simulink model "LoFT_Example3"  (R2024b)
settings: Solver=ode4  StartTime=0.0  StopTime=300  FixedStep=simu.dt  RelTol=1e-3
undefined symbols (not defined in the file): body, circtime, Communication, D1, Delta, irkb, line, LoFT, p0, Pn, s, simu, trip_time, Turbwind, waves, wind
libraries: simulink x350, spsThreePhaseVIMeasurementLib x41, spsThreePhasePISectionLineLib x34, spsThreePhaseParallelRLCLoadLib x21, spsThreePhaseTransformerTwoWindingsLib x14, spsLoadFlowBusLib x10, spsThreePhaseDynamicLoadLib x9, spsSynchronousMachinepuStandardLib x7, spsExcitationSystemLib x7, spsSteamTurbineandGovernorLib x7, spsGenericPowerSystemStabilizerLib x7, spsMultiBandPowerSystemStabilizerLib x7
(part 38 of 49)

== system LoFT_Example3/FOWT System/Subsystem7/FOWT8/Hydrodynamics/excitation force ==
  position : Inport
  Wave : Inport  Port=2
  Clock : Clock  Commented=on
  Frequency Spacing Delta Omega : Constant  Commented=on  Value=waves.dOmega/10  VectorParams1D=off
  Imaginary Part of Wave Excitation : Constant  Commented=on  Value=body.hydroForce.fExt.im(:,:,[1,3,5])  VectorParams1D=off
  Random Phase : Constant  Commented=on  Value=waves.phase  VectorParams1D=off
  Real Part of Wave Excitation : Constant  Commented=on  Value=body.hydroForce.fExt.re(:,:,[1,3,5])  VectorParams1D=off
  Real Part of Wave Excitation1 : Constant  Commented=on  Value=body.hydroForce.fExt.md(:,:,[1,3,5])  VectorParams1D=off
  WECSim Linear wave excitiation : MATLAB Function  Commented=on  TreatAsAtomicUnit=on
  Wave Frequency : Constant  Commented=on  Value=waves.omega/10  VectorParams1D=off
  Wave Spectrum : Constant  Commented=on  Value=waves.amplitude  VectorParams1D=off
  Wave direction spread : Constant  Commented=on  Value=waves.spread  VectorParams1D=off
  Wave direction1 : Constant  Commented=on  Value=waves.direction  VectorParams1D=off
  Fext : Outport
  wires:
  Wave/1 -> Fext/1
  Wave direction1/1 -> WECSim Linear wave excitiation/8(WaveDir)
  Frequency Spacing Delta Omega/1 -> WECSim Linear wave excitiation/6(dw)
  Wave Spectrum/1 -> WECSim Linear wave excitiation/1(A)
  Imaginary Part of Wave Excitation/1 -> WECSim Linear wave excitiation/4(fExtIM)
  Random Phase/1 -> WECSim Linear wave excitiation/5(phaseRand)
  Wave Frequency/1 -> WECSim Linear wave excitiation/2(w)
  Real Part of Wave Excitation1/1 -> WECSim Linear wave excitiation/10(fExtMD)
  Wave direction spread/1 -> WECSim Linear wave excitiation/9(spread)
  Clock/1 -> WECSim Linear wave excitiation/7(time)
  Real Part of Wave Excitation/1 -> WECSim Linear wave excitiation/3(fExtRE)

== system LoFT_Example3/FOWT System/Subsystem7/FOWT8/Hydrodynamics/radiation force ==
  velocity : Inport
  In2 : Inport  Port=2
  Add : Sum
  Constant1 : Constant  Value=Hydro.radiationaddedmass
  Constant2 : Constant  Value=Hydro.radiationdamping
  Demux : Demux  Commented=on  Outputs=3
  Demux1 : Demux  Commented=on  Outputs=3
  Gain : Gain  Commented=on  Gain=-1
  IRBK : Constant  Commented=on  Value=irkb(:,[1,3,5],[[1,3,5]])
  MATLAB Function : MATLAB Function  Commented=on  TreatAsAtomicUnit=on
  Product : Product  Multiplication=Matrix(*)
  Product1 : Product  Multiplication=Matrix(*)
  Rate Transition : RateTransition  Commented=on
  Reshape : Reshape  Commented=on
  Scope1 : Scope  Commented=on  NumInputPorts=2
  Scope2 : Scope  Commented=on  NumInputPorts=2
  Scope3 : Scope  Commented=on  NumInputPorts=2
  cicTime : Constant  Commented=on  Value=circtime
  F_rad : Outport
  wires:
  Add/1 -> F_rad/1
  Product/1 -> Add/1
  Constant2/1 -> Product1/1
  Constant1/1 -> Product/1
  In2/1 -> MATLAB Function/1(velocity), Product1/2
  IRBK/1 -> MATLAB Function/2(irkb)
  Rate Transition/1 -> Reshape/1
  cicTime/1 -> MATLAB Function/3(circtime)
  MATLAB Function/1(radiationdamping) -> Rate Transition/1
  velocity/1 -> Product/2
  Reshape/1 -> Gain/1
  Demux1/1 -> Scope1/1
  Demux/1 -> Scope1/2
  Demux1/2 -> Scope2/1
  Demux/2 -> Scope2/2
  Demux1/3 -> Scope3/1
  Demux/3 -> Scope3/2
  Gain/1 -> Demux/1
  Product1/1 -> Demux1/1, Add/2

== system LoFT_Example3/FOWT System/Subsystem7/FOWT8/Hydrodynamics/viscous force  ==
  In1 : Inport
  Abs : Abs  SaturateOnIntegerOverflow=off
  Constant3 : Constant  Value=Hydro.viscious
  Product2 : Product  Multiplication=Matrix(*)
  Product3 : Product
  F_vis : Outport
  wires:
  Product2/1 -> F_vis/1
  Product3/1 -> Product2/2
  In1/1 -> Product3/2, Abs/1
  Constant3/1 -> Product2/1
  Abs/1 -> Product3/1

== system LoFT_Example3/FOWT System/Subsystem7/FOWT8/wind speed(m//s)/smooth1 ==
  In1 : Inport
  Gain : Gain
  Gain1 : Gain
  Integrator : Integrator
  Scope : Scope  NumInputPorts=2
  Sum : Sum  Inputs=|+-
  FB : Outport
  wires:
  Gain1/1 -> Scope/2, FB/1
  Integrator/1 -> Gain1/1, Gain/1
  Sum/1 -> Integrator/1
  Gain/1 -> Sum/2
  In1/1 -> Scope/1, Sum/1

== system LoFT_Example3/FOWT System/Subsystem7/FOWT9/Aerodynamics and Local Control Systems/Hull Aerodynamic ==
  In1 : Inport
  In2 : Inport  Port=2
  In4 : Inport  Port=3
  2-D Lookup Table1 : Lookup_n-D  BreakpointsForDimension1=Aero.TSR(1:1:24)  BreakpointsForDimension2=Aero.BlPitch(6:1:36)  Table=max(Aero.Ctmat(1:24,6:36),0)  InternalRulePriority=Speed  RndMeth=Simplest
      settings: InputPortMap=u0,u1
  Add1 : Sum
  Constant : Constant  Value=0
  Divide2 : Product  Inputs=*/
  Gain1 : Gain  Gain=0.5*1.225*pi*120^2*0.975*1.1
  Gain3 : Gain  Gain=120
  Gain5 : Gain  Gain=180/pi
  Product2 : Product
  Product3 : Product
  Saturation1 : Saturate  UpperLimit=2  LowerLimit=0
  Tower : Gain  Gain=0.613 * Aero.Cs * Aero.Ch * Aero.S
  Transfer Fcn2 : TransferFcn  Denominator=[0.2 1]
  Vector Concatenate1 : Concatenate  NumInputs=3
  mean force arm : Gain  Gain=92.8
  Out1 : Outport
  Rotor thrust : Outport  Port=2
  wires:
  Vector Concatenate1/1 -> Out1/1
  In4/1 -> Gain5/1
  In2/1 -> Gain3/1
  mean force arm/1 -> Vector Concatenate1/3
  Gain1/1 -> Product3/2
  Gain5/1 -> 2-D Lookup Table1/2
  Gain3/1 -> Divide2/1
  Divide2/1 -> 2-D Lookup Table1/1
  Product2/1 -> Product3/1, Tower/1
  Transfer Fcn2/1 -> Add1/2
  Constant/1 -> Vector Concatenate1/2
  Add1/1 -> mean force arm/1, Vector Concatenate1/1, Rotor thrust/1
  Saturation1/1 -> Gain1/1
  2-D Lookup Table1/1 -> Saturation1/1
  Product3/1 -> Transfer Fcn2/1
  In1/1 -> Divide2/2, Product2/1, Product2/2
  Tower/1 -> Add1/1

== system LoFT_Example3/FOWT System/Subsystem7/FOWT9/Aerodynamics and Local Control Systems/Local Control Systems ==
  WindSpeed : Inport
  RotSpeed : Inport  Port=2
  Nacelle Speed : Inport  Port=3
  " " : StateSpace  A=Controller.omegaFilter.A  B=Controller.omegaFilter.B  C=Controller.omegaFilter.C  D=Controller.omegaFilter.D  InitialCondition=[0,(7.55*pi/30)/Controller.omegaFilter.C(2)]
  Delay : Delay  DelayLength=1  InitialCondition=0
  Subsystem : Subsystem
  Subsystem1 : Subsystem
  Subsystem2 : Subsystem
  Transfer Fcn : TransferFcn  Denominator="[Controller.pitchFilter.A,   Controller.pitchFilter.B    1]"
  wind speed estimator : Subsystem
  GenTorq : Outport
  BldPitch : Outport  Port=2
  wires:
  wind speed estimator/1(Out1) -> Subsystem1/2(WindSpeed), Subsystem/1(WindSpeed)
  Delay/1 -> Subsystem1/3(3), Subsystem/2(2)
  [Delta_omega_g] -> Delay/1
  Subsystem/1(GenTorq) -> GenTorq/1, Subsystem2/1(GenTorq)
  Subsystem1/1(BldPitch) -> Subsystem2/2(BldPitch), BldPitch/1
  Subsystem2/1(Delta_omega_g) -> [Delta_omega_g]
  RotSpeed/1 -> " "/1
  Nacelle Speed/1 -> Transfer Fcn/1
  Transfer Fcn/1 -> Subsystem1/4(Nacelle Speed)
  " "/1 -> Subsystem1/1(RotSpeed), Subsystem/3(RotSpeed)
  WindSpeed/1 -> wind speed estimator/1(In1)

== system LoFT_Example3/FOWT System/Subsystem7/FOWT9/Aerodynamics and Local Control Systems/Rotor//drivetrain dynamics ==
  In1 : Inport
  In2 : Inport  Port=2
  In3 : Inport  Port=3
  In4 : Inport  Port=4
  In5 : Inport  Port=5
  1/J_rot : Gain  Gain=1/(LoFT.Property.rotorinertia)
  2-D Lookup Table : Lookup_n-D  BreakpointsForDimension1=Aero.TSR(1:1:24)  BreakpointsForDimension2=Aero.BlPitch(6:1:36)  Table=max(Aero.Cpmat(1:24,6:36),0)  InternalRulePriority=Speed  RndMeth=Simplest
      settings: InputPortMap=u0,u1
  Divide : Product  Inputs=**/
  Divide1 : Product  Inputs=*/
  Gain : Gain  Gain=0.5 * 1.225 * pi * 120^2 * 0.965 * 0.975
  Gain2 : Gain  Gain=120
  Gain4 : Gain  Gain=180/pi
  Integrator : Integrator  InitialCondition=Initstate(1)
  Product1 : Product  Inputs=3
  Saturation : Saturate  UpperLimit=1  LowerLimit=0
  Saturation3 : Saturate  UpperLimit=1.5  LowerLimit=0.3
  Sum : Sum  Inputs=|+-
  Transfer Fcn1 : TransferFcn  Denominator=[0.2 1]
  Out1 : Outport
  Out2 : Outport  Port=2
  wires:
  In1/1 -> Gain2/1
  In2/1 -> Divide1/2
  Sum/1 -> Transfer Fcn1/1
  In5/1 -> Sum/2
  Product1/1 -> Divide/2
  Gain2/1 -> Divide1/1
  Gain/1 -> Divide/1
  1/J_rot/1 -> Integrator/1
  Integrator/1 -> Saturation3/1
  In3/1 -> Gain4/1
  Transfer Fcn1/1 -> 1/J_rot/1
  2-D Lookup Table/1 -> Saturation/1
  Gain4/1 -> 2-D Lookup Table/2
  In4/1 -> Product1/1, Product1/2, Product1/3
  Saturation/1 -> Gain/1
  Divide1/1 -> 2-D Lookup Table/1
  Divide/1 -> Sum/1, Out2/1
  Saturation3/1 -> Divide/3, Out1/1

== system LoFT_Example3/FOWT System/Subsystem7/FOWT9/Aerodynamics and Local Control Systems/smooth1 ==
  In1 : Inport
  Gain : Gain  Gain=10
  Gain1 : Gain  Gain=10
  Integrator : Integrator  InitialCondition=0.1*8e6
  Scope : Scope  NumInputPorts=2
  Sum : Sum  Inputs=|+-
  Out1 : Outport
  wires:
  In1/1 -> Sum/1, Scope/1
  Gain/1 -> Sum/2
  Sum/1 -> Integrator/1
  Integrator/1 -> Gain/1, Gain1/1
  Gain1/1 -> Out1/1, Scope/2

== system LoFT_Example3/FOWT System/Subsystem7/FOWT9/Aerodynamics and Local Control Systems/wind speed estimator ==
  In1 : Inport
  Discrete Filter : DiscreteFilter  Numerator=Controller.F.Wind.b  Denominator=Controller.F.Wind.a  InitialStates=2000
  Out1 : Outport
  wires:
  Discrete Filter/1 -> Out1/1
  In1/1 -> Discrete Filter/1

== system LoFT_Example3/FOWT System/Subsystem7/FOWT9/Hydrodynamics/excitation force ==
  position : Inport
  Wave : Inport  Port=2
  Clock : Clock  Commented=on
  Frequency Spacing Delta Omega : Constant  Commented=on  Value=waves.dOmega/10  VectorParams1D=off
  Imaginary Part of Wave Excitation : Constant  Commented=on  Value=body.hydroForce.fExt.im(:,:,[1,3,5])  VectorParams1D=off
  Random Phase : Constant  Commented=on  Value=waves.phase  VectorParams1D=off
  Real Part of Wave Excitation : Constant  Commented=on  Value=body.hydroForce.fExt.re(:,:,[1,3,5])  VectorParams1D=off
  Real Part of Wave Excitation1 : Constant  Commented=on  Value=body.hydroForce.fExt.md(:,:,[1,3,5])  VectorParams1D=off
  WECSim Linear wave excitiation : MATLAB Function  Commented=on  TreatAsAtomicUnit=on
  Wave Frequency : Constant  Commented=on  Value=waves.omega/10  VectorParams1D=off
  Wave Spectrum : Constant  Commented=on  Value=waves.amplitude  VectorParams1D=off
  Wave direction spread : Constant  Commented=on  Value=waves.spread  VectorParams1D=off
  Wave direction1 : Constant  Commented=on  Value=waves.direction  VectorParams1D=off
  Fext : Outport
  wires:
  Real Part of Wave Excitation/1 -> WECSim Linear wave excitiation/3(fExtRE)
  Clock/1 -> WECSim Linear wave excitiation/7(time)
  Wave direction spread/1 -> WECSim Linear wave excitiation/9(spread)
  Real Part of Wave Excitation1/1 -> WECSim Linear wave excitiation/10(fExtMD)
  Wave Frequency/1 -> WECSim Linear wave excitiation/2(w)
  Random Phase/1 -> WECSim Linear wave excitiation/5(phaseRand)
  Imaginary Part of Wave Excitation/1 -> WECSim Linear wave excitiation/4(fExtIM)
  Wave Spectrum/1 -> WECSim Linear wave excitiation/1(A)
  Frequency Spacing Delta Omega/1 -> WECSim Linear wave excitiation/6(dw)
  Wave direction1/1 -> WECSim Linear wave excitiation/8(WaveDir)
  Wave/1 -> Fext/1

== system LoFT_Example3/FOWT System/Subsystem7/FOWT9/Hydrodynamics/radiation force ==
  velocity : Inport
  In2 : Inport  Port=2
  Add : Sum
  Constant1 : Constant  Value=Hydro.radiationaddedmass
  Constant2 : Constant  Value=Hydro.radiationdamping
  Demux : Demux  Commented=on  Outputs=3
  Demux1 : Demux  Commented=on  Outputs=3
  Gain : Gain  Commented=on  Gain=-1
  IRBK : Constant  Commented=on  Value=irkb(:,[1,3,5],[[1,3,5]])
  MATLAB Function : MATLAB Function  Commented=on  TreatAsAtomicUnit=on
  Product : Product  Multiplication=Matrix(*)
  Product1 : Product  Multiplication=Matrix(*)
  Rate Transition : RateTransition  Commented=on
  Reshape : Reshape  Commented=on
  Scope1 : Scope  Commented=on  NumInputPorts=2
  Scope2 : Scope  Commented=on  NumInputPorts=2
  Scope3 : Scope  Commented=on  NumInputPorts=2
  cicTime : Constant  Commented=on  Value=circtime
  F_rad : Outport
  wires:
  Product1/1 -> Add/2, Demux1/1
  Gain/1 -> Demux/1
  Demux/3 -> Scope3/2
  Demux1/3 -> Scope3/1
  Demux/2 -> Scope2/2
  Demux1/2 -> Scope2/1
  Demux/1 -> Scope1/2
  Demux1/1 -> Scope1/1
  Reshape/1 -> Gain/1
  velocity/1 -> Product/2
  MATLAB Function/1(radiationdamping) -> Rate Transition/1
  cicTime/1 -> MATLAB Function/3(circtime)
  Rate Transition/1 -> Reshape/1
  IRBK/1 -> MATLAB Function/2(irkb)
  In2/1 -> Product1/2, MATLAB Function/1(velocity)
  Constant1/1 -> Product/1
  Constant2/1 -> Product1/1
  Product/1 -> Add/1
  Add/1 -> F_rad/1

== system LoFT_Example3/FOWT System/Subsystem7/FOWT9/Hydrodynamics/viscous force  ==
  In1 : Inport
  Abs : Abs  SaturateOnIntegerOverflow=off
  Constant3 : Constant  Value=Hydro.viscious
  Product2 : Product  Multiplication=Matrix(*)
  Product3 : Product
  F_vis : Outport
  wires:
  Abs/1 -> Product3/1
  Constant3/1 -> Product2/1
  In1/1 -> Abs/1, Product3/2
  Product3/1 -> Product2/2
  Product2/1 -> F_vis/1

== system LoFT_Example3/FOWT System/Subsystem7/FOWT9/wind speed(m//s)/smooth1 ==
  In1 : Inport
  Gain : Gain
  Gain1 : Gain
  Integrator : Integrator
  Scope : Scope  NumInputPorts=2
  Sum : Sum  Inputs=|+-
  FB : Outport
  wires:
  In1/1 -> Sum/1, Scope/1
  Gain/1 -> Sum/2
  Sum/1 -> Integrator/1
  Integrator/1 -> Gain/1, Gain1/1
  Gain1/1 -> FB/1, Scope/2

== system LoFT_Example3/Onshore grid/Onshore Grid/Subsystem/SG1/Regulators1 ==
  m : Inport
  Bus Selector1 : BusSelector  OutputSignals="dq0 components.Stator voltage  vq (pu),dq0 components.Stator voltage  vd (pu),Mechanical.Rotor speed  wm  (pu),Output active power   Peo (pu)"
  Math Function1 : Math  Operator=hypot  SignedPower=on
  Pref1 : Constant
  Scope : Scope
  Turbine  & Excitation Regulators Mac2 : Subsystem
  Vref : Constant
  Pm : Outport  VectorParamsAs1DForOutWhenUnconnected=off
  Vf : Outport  Port=2  VectorParamsAs1DForOutWhenUnconnected=off
  wires:
  m/1 -> Bus Selector1/1
  Bus Selector1/4 -> Turbine  & Excitation Regulators Mac2/6(Pe)  "<Output active power   Peo (pu)>"
  Bus Selector1/3 -> Turbine  & Excitation Regulators Mac2/5(w)  "<Rotor speed  wm  (pu)>"
  Bus Selector1/2 -> Turbine  & Excitation Regulators Mac2/3(Vd), Math Function1/2  "<Stator voltage  vd (pu)>"
  Bus Selector1/1 -> Turbine  & Excitation Regulators Mac2/4(Vq), Math Function1/1  "<Stator voltage  vq (pu)>"
  Turbine  & Excitation Regulators Mac2/2(Vf) -> Vf/1
  Vref/1 -> Turbine  & Excitation Regulators Mac2/1(Pref)
  Turbine  & Excitation Regulators Mac2/1(Pm) -> Pm/1
  Pref1/1 -> Turbine  & Excitation Regulators Mac2/2(Vref)
  Math Function1/1 -> Scope/1

== system LoFT_Example3/Onshore grid/Onshore Grid/Subsystem/SG2/Regulators2 ==
  m : Inport
  Bus Selector1 : BusSelector  OutputSignals="dq0 components.Stator voltage  vq (pu),dq0 components.Stator voltage  vd (pu),Mechanical.Rotor speed  wm  (pu),Output active power   Peo (pu)"
  Math Function1 : Math  Operator=hypot  SignedPower=on
  Pref1 : Constant
  Scope : Scope
  Turbine  & Excitation Regulators Mac2 : Subsystem
  Vref : Constant  Value=0.52081
  Pm : Outport  VectorParamsAs1DForOutWhenUnconnected=off
  Vf : Outport  Port=2  VectorParamsAs1DForOutWhenUnconnected=off
  wires:
  m/1 -> Bus Selector1/1
  Bus Selector1/4 -> Turbine  & Excitation Regulators Mac2/6(Pe)  "<Output active power   Peo (pu)>"
  Bus Selector1/3 -> Turbine  & Excitation Regulators Mac2/5(w)  "<Rotor speed  wm  (pu)>"
  Bus Selector1/2 -> Turbine  & Excitation Regulators Mac2/3(Vd), Math Function1/2  "<Stator voltage  vd (pu)>"
  Bus Selector1/1 -> Turbine  & Excitation Regulators Mac2/4(Vq), Math Function1/1  "<Stator voltage  vq (pu)>"
  Turbine  & Excitation Regulators Mac2/2(Vf) -> Vf/1
  Vref/1 -> Turbine  & Excitation Regulators Mac2/1(Pref)
  Turbine  & Excitation Regulators Mac2/1(Pm) -> Pm/1
  Pref1/1 -> Turbine  & Excitation Regulators Mac2/2(Vref)
  Math Function1/1 -> Scope/1

== system LoFT_Example3/Onshore grid/Onshore Grid/Subsystem/SG4/Regulators4 ==
  m : Inport
  Bus Selector1 : BusSelector  OutputSignals="dq0 components.Stator voltage  vq (pu),dq0 components.Stator voltage  vd (pu),Mechanical.Rotor speed  wm  (pu),Output active power   Peo (pu)"
  Math Function1 : Math  Operator=hypot  SignedPower=on
  Pref1 : Constant
  Scope : Scope
  Turbine  & Excitation Regulators Mac2 : Subsystem
  Vref : Constant  Value=0.632
  Pm : Outport  VectorParamsAs1DForOutWhenUnconnected=off
  Vf : Outport  Port=2  VectorParamsAs1DForOutWhenUnconnected=off
  wires:
  m/1 -> Bus Selector1/1
  Bus Selector1/4 -> Turbine  & Excitation Regulators Mac2/6(Pe)  "<Output active power   Peo (pu)>"
  Bus Selector1/3 -> Turbine  & Excitation Regulators Mac2/5(w)  "<Rotor speed  wm  (pu)>"
  Bus Selector1/2 -> Turbine  & Excitation Regulators Mac2/3(Vd), Math Function1/2  "<Stator voltage  vd (pu)>"
  Bus Selector1/1 -> Turbine  & Excitation Regulators Mac2/4(Vq), Math Function1/1  "<Stator voltage  vq (pu)>"
  Turbine  & Excitation Regulators Mac2/2(Vf) -> Vf/1
  Vref/1 -> Turbine  & Excitation Regulators Mac2/1(Pref)
  Turbine  & Excitation Regulators Mac2/1(Pm) -> Pm/1
  Pref1/1 -> Turbine  & Excitation Regulators Mac2/2(Vref)
  Math Function1/1 -> Scope/1

== system LoFT_Example3/Onshore grid/Onshore Grid/Subsystem/SG5/Regulators5 ==
  m : Inport
  Bus Selector1 : BusSelector  OutputSignals="dq0 components.Stator voltage  vq (pu),dq0 components.Stator voltage  vd (pu),Mechanical.Rotor speed  wm  (pu),Output active power   Peo (pu)"
  Math Function1 : Math  Operator=hypot  SignedPower=on
  Pref1 : Constant
  Scope : Scope
  Turbine  & Excitation Regulators Mac2 : Subsystem
  Vref : Constant  Value=0.508
  Pm : Outport  VectorParamsAs1DForOutWhenUnconnected=off
  Vf : Outport  Port=2  VectorParamsAs1DForOutWhenUnconnected=off
  wires:
  m/1 -> Bus Selector1/1
  Bus Selector1/4 -> Turbine  & Excitation Regulators Mac2/6(Pe)  "<Output active power   Peo (pu)>"
  Bus Selector1/3 -> Turbine  & Excitation Regulators Mac2/5(w)  "<Rotor speed  wm  (pu)>"
  Math Function1/1 -> Scope/1
  Bus Selector1/2 -> Turbine  & Excitation Regulators Mac2/3(Vd), Math Function1/2  "<Stator voltage  vd (pu)>"
  Bus Selector1/1 -> Turbine  & Excitation Regulators Mac2/4(Vq), Math Function1/1  "<Stator voltage  vq (pu)>"
  Turbine  & Excitation Regulators Mac2/2(Vf) -> Vf/1
  Vref/1 -> Turbine  & Excitation Regulators Mac2/1(Pref)
  Turbine  & Excitation Regulators Mac2/1(Pm) -> Pm/1
  Pref1/1 -> Turbine  & Excitation Regulators Mac2/2(Vref)

== system LoFT_Example3/Onshore grid/Onshore Grid/Subsystem/SG6/Regulators6 ==
  m : Inport
  Bus Selector1 : BusSelector  OutputSignals="dq0 components.Stator voltage  vq (pu),dq0 components.Stator voltage  vd (pu),Mechanical.Rotor speed  wm  (pu),Output active power   Peo (pu)"
  Math Function1 : Math  Operator=hypot  SignedPower=on
  Pref1 : Constant
  Scope : Scope
  Turbine  & Excitation Regulators Mac2 : Subsystem
  Vref : Constant  Value=0.65
  Pm : Outport  VectorParamsAs1DForOutWhenUnconnected=off
  Vf : Outport  Port=2  VectorParamsAs1DForOutWhenUnconnected=off
  wires:
  m/1 -> Bus Selector1/1
  Bus Selector1/4 -> Turbine  & Excitation Regulators Mac2/6(Pe)  "<Output active power   Peo (pu)>"
  Bus Selector1/3 -> Turbine  & Excitation Regulators Mac2/5(w)  "<Rotor speed  wm  (pu)>"
  Bus Selector1/2 -> Turbine  & Excitation Regulators Mac2/3(Vd), Math Function1/2  "<Stator voltage  vd (pu)>"
  Bus Selector1/1 -> Turbine  & Excitation Regulators Mac2/4(Vq), Math Function1/1  "<Stator voltage  vq (pu)>"
  Turbine  & Excitation Regulators Mac2/2(Vf) -> Vf/1
  Vref/1 -> Turbine  & Excitation Regulators Mac2/1(Pref)
  Turbine  & Excitation Regulators Mac2/1(Pm) -> Pm/1
  Pref1/1 -> Turbine  & Excitation Regulators Mac2/2(Vref)
  Math Function1/1 -> Scope/1

== system LoFT_Example3/Onshore grid/Onshore Grid/Subsystem/SG8/Regulators8 ==
  m : Inport
  Bus Selector1 : BusSelector  OutputSignals="dq0 components.Stator voltage  vq (pu),dq0 components.Stator voltage  vd (pu),Mechanical.Rotor speed  wm  (pu),Output active power   Peo (pu)"
  Math Function1 : Math  Operator=hypot  SignedPower=on
  Pref1 : Constant
  Scope : Scope
  Turbine  & Excitation Regulators Mac2 : Subsystem
  Vref : Constant  Value=0.54
  Pm : Outport  VectorParamsAs1DForOutWhenUnconnected=off
  Vf : Outport  Port=2  VectorParamsAs1DForOutWhenUnconnected=off
  wires:
  m/1 -> Bus Selector1/1
  Bus Selector1/4 -> Turbine  & Excitation Regulators Mac2/6(Pe)  "<Output active power   Peo (pu)>"
  Bus Selector1/3 -> Turbine  & Excitation Regulators Mac2/5(w)  "<Rotor speed  wm  (pu)>"
  Bus Selector1/2 -> Turbine  & Excitation Regulators Mac2/3(Vd), Math Function1/2  "<Stator voltage  vd (pu)>"
  Bus Selector1/1 -> Turbine  & Excitation Regulators Mac2/4(Vq), Math Function1/1  "<Stator voltage  vq (pu)>"
  Turbine  & Excitation Regulators Mac2/2(Vf) -> Vf/1
  Vref/1 -> Turbine  & Excitation Regulators Mac2/1(Pref)
  Turbine  & Excitation Regulators Mac2/1(Pm) -> Pm/1
  Pref1/1 -> Turbine  & Excitation Regulators Mac2/2(Vref)
  Math Function1/1 -> Scope/1

== system LoFT_Example3/Onshore grid/Onshore Grid/Subsystem/SG9/Regulators9 ==
  m : Inport
  Bus Selector1 : BusSelector  OutputSignals="dq0 components.Stator voltage  vq (pu),dq0 components.Stator voltage  vd (pu),Mechanical.Rotor speed  wm  (pu),Output active power   Peo (pu)"
  Math Function1 : Math  Operator=hypot  SignedPower=on
  Pref1 : Constant
  Scope : Scope
  Turbine  & Excitation Regulators Mac2 : Subsystem
  Vref : Constant  Value=0.83
  Pm : Outport  VectorParamsAs1DForOutWhenUnconnected=off
  Vf : Outport  Port=2  VectorParamsAs1DForOutWhenUnconnected=off
  wires:
  m/1 -> Bus Selector1/1
  Bus Selector1/4 -> Turbine  & Excitation Regulators Mac2/6(Pe)  "<Output active power   Peo (pu)>"
  Bus Selector1/3 -> Turbine  & Excitation Regulators Mac2/5(w)  "<Rotor speed  wm  (pu)>"
  Bus Selector1/2 -> Turbine  & Excitation Regulators Mac2/3(Vd), Math Function1/2  "<Stator voltage  vd (pu)>"
  Bus Selector1/1 -> Turbine  & Excitation Regulators Mac2/4(Vq), Math Function1/1  "<Stator voltage  vq (pu)>"
  Turbine  & Excitation Regulators Mac2/2(Vf) -> Vf/1
  Vref/1 -> Turbine  & Excitation Regulators Mac2/1(Pref)
  Turbine  & Excitation Regulators Mac2/1(Pm) -> Pm/1
  Pref1/1 -> Turbine  & Excitation Regulators Mac2/2(Vref)
  Math Function1/1 -> Scope/1

== system LoFT_Example3/FOWT System/Subsystem1/FOWT1/Aerodynamics and Local Control Systems/Local Control Systems/Subsystem ==
  WindSpeed : Inport
  2 : Inport  Port=2
  RotSpeed : Inport  Port=3
  Compare To Constant1 : simulink/Logic and Bit Operations/Compare To Constant  relop=>=  const=0  OutDataTypeStr=boolean
  Divide4 : Product  Inputs=**
  Gain5 : Gain  Gain=Controller.R.VS_KI
  Gain6 : Gain  Gain=Controller.R.VS_KP
  Integrator1 : Integrator  InitialCondition=Controller.torqueMax * 0.7  LimitOutput=on  UpperSaturationLimit=Controller.torqueMax
  Optimall TSR / Radius : Gain  Gain=Controller.R.VS_TSRopt/Controller.R.RotorRad
  Rate Limiter : RateLimiter  RisingSlewLimit=Controller.torqueMaxRate  FallingSlewLimit=-Controller.torqueMaxRate  SampleTimeMode=inherited
  Saturation : Saturate  UpperLimit=7.55*pi/30  LowerLimit=5*pi/30
  Saturation1 : Saturate  UpperLimit=Controller.torqueMax  LowerLimit=0
  Saturation2 : Saturate  UpperLimit=7.55*pi/30  LowerLimit=5*pi/30
  Scope2 : Scope
  Sum2 : Sum  Inputs=|+-
  Sum7 : Sum  Inputs=|+-
  Sum8 : Sum  Inputs=|++
  GenTorq : Outport
  wires:
  Gain6/1 -> Sum8/1
  WindSpeed/1 -> Optimall TSR / Radius/1
  Sum7/1 -> Saturation/1
  Divide4/1 -> Scope2/1, Sum7/2
  2/1 -> Compare To Constant1/1, Divide4/2
  Rate Limiter/1 -> GenTorq/1
  Saturation/1 -> Sum2/1
  Compare To Constant1/1 -> Divide4/1
  Sum2/1 -> Gain6/1, Gain5/1
  Integrator1/1 -> Sum8/2
  Gain5/1 -> Integrator1/1
  Sum8/1 -> Saturation1/1
  RotSpeed/1 -> Sum2/2
  Saturation1/1 -> Rate Limiter/1
  Saturation2/1 -> Sum7/1
  Optimall TSR / Radius/1 -> Saturation2/1

== system LoFT_Example3/FOWT System/Subsystem1/FOWT1/Aerodynamics and Local Control Systems/Local Control Systems/Subsystem1 ==
  RotSpeed : Inport
  WindSpeed : Inport  Port=2
  3 : Inport  Port=3
  Nacelle Speed : Inport  Port=4
  1-D Lookup Table : Lookup_n-D  NumberOfTableDimensions=1  BreakpointsForDimension1=Controller.R.PS_WindSpeeds  Table=Controller.R.PS_BldPitchMin  InternalRulePriority=Speed  RndMeth=Simplest
  Compare To Constant : simulink/Logic and Bit Operations/Compare To Constant  relop=<=  const=0  OutDataTypeStr=boolean
  Constant : Constant  Value=7.55*pi/30
  Constant1 : Constant  Value=90*pi/180
  Delay : Delay  DelayLength=1  InitialCondition=0
  Divide3 : Product  Inputs=**
  Gain : Gain  Gain=Controller.KV *0.5
  Gain Scheduling : Subsystem
  Gain1 : Gain
  Rate Limiter : RateLimiter  RisingSlewLimit=2*pi/180  FallingSlewLimit=-2 * pi/180  SampleTimeMode=inherited
  Saturation : Saturate  UpperLimit=7.55*pi/30  LowerLimit=5*pi/30
  Saturation Dynamic : simulink/Discontinuities/Saturation Dynamic  OutMin=[]  OutMax=[]  OutDataTypeStr=Inherit: Same as second input  OutDataType=fixdt(1, 16)  OutScaling=2^-10  DoSatur=off
  Scope2 : Scope
  Sum1 : Sum  Inputs=|++
  Sum3 : Sum  Inputs=|+-
  Sum4 : Sum  Inputs=|+-
  BldPitch : Outport
  wires:
  Saturation/1 -> Sum3/1
  Sum4/1 -> Saturation/1
  Rate Limiter/1 -> BldPitch/1
  Gain1/1 -> Scope2/1, Gain Scheduling/2(In3), Saturation Dynamic/3
  1-D Lookup Table/1 -> Gain1/1
  WindSpeed/1 -> 1-D Lookup Table/1  "Vhat"
  Nacelle Speed/1 -> Gain/1
  Gain/1 -> Sum1/2
  Sum1/1 -> Saturation Dynamic/2
  Gain Scheduling/1(Out1) -> Sum1/1
  RotSpeed/1 -> Sum3/2
  Delay/1 -> Gain Scheduling/3(In2)
  3/1 -> Divide3/2, Compare To Constant/1
  Constant1/1 -> Saturation Dynamic/1
  Constant/1 -> Sum4/1
  Compare To Constant/1 -> Divide3/1
  Saturation Dynamic/1 -> Delay/1, Rate Limiter/1
  Sum3/1 -> Gain Scheduling/1(In1)
  Divide3/1 -> Sum4/2

== system LoFT_Example3/FOWT System/Subsystem1/FOWT1/Aerodynamics and Local Control Systems/Local Control Systems/Subsystem2 ==
  GenTorq : Inport
  BldPitch : Inport  Port=2
  Constant3 : Constant  Value=-Controller.torqueMax
  Gain 1 : Gain  Gain=Controller.SPS_kb/deg2rad(30)
  Gain 2 : Gain  Gain=Controller.omegaMax
  Gain 3 : Gain  Gain=-Controller.SPS_kt/Controller.torqueMax
  Sum5 : Sum  Inputs=|+-
  Sum6 : Sum  Inputs=|+-
  Delta_omega_g : Outport
  wires:
  GenTorq/1 -> Sum5/1
  BldPitch/1 -> Gain 1/1
  Gain 2/1 -> Delta_omega_g/1
  Sum5/1 -> Gain 3/1
  Gain 3/1 -> Sum6/2
  Constant3/1 -> Sum5/2
  Gain 1/1 -> Sum6/1
  Sum6/1 -> Gain 2/1

== system LoFT_Example3/FOWT System/Subsystem1/FOWT1/Aerodynamics and Local Control Systems/Local Control Systems/wind speed estimator ==
  In1 : Inport
  Discrete Filter : DiscreteFilter  Numerator=Controller.F.Wind.b  Denominator=Controller.F.Wind.a  InitialStates=2000
  Out1 : Outport
  wires:
  In1/1 -> Discrete Filter/1
  Discrete Filter/1 -> Out1/1

== system LoFT_Example3/FOWT System/Subsystem1/FOWT10/Aerodynamics and Local Control Systems/Local Control Systems/Subsystem ==
  WindSpeed : Inport
  2 : Inport  Port=2
  RotSpeed : Inport  Port=3
  Compare To Constant1 : simulink/Logic and Bit Operations/Compare To Constant  relop=>=  const=0  OutDataTypeStr=boolean
  Divide4 : Product  Inputs=**
  Gain5 : Gain  Gain=Controller.R.VS_KI
  Gain6 : Gain  Gain=Controller.R.VS_KP
  Integrator1 : Integrator  InitialCondition=Controller.torqueMax * 0.7  LimitOutput=on  UpperSaturationLimit=Controller.torqueMax
  Optimall TSR / Radius : Gain  Gain=Controller.R.VS_TSRopt/Controller.R.RotorRad
  Rate Limiter : RateLimiter  RisingSlewLimit=Controller.torqueMaxRate  FallingSlewLimit=-Controller.torqueMaxRate  SampleTimeMode=inherited
  Saturation : Saturate  UpperLimit=7.55*pi/30  LowerLimit=5*pi/30
  Saturation1 : Saturate  UpperLimit=Controller.torqueMax  LowerLimit=0
  Saturation2 : Saturate  UpperLimit=7.55*pi/30  LowerLimit=5*pi/30
  Scope2 : Scope
  Sum2 : Sum  Inputs=|+-
  Sum7 : Sum  Inputs=|+-
  Sum8 : Sum  Inputs=|++
  GenTorq : Outport
  wires:
  Optimall TSR / Radius/1 -> Saturation2/1
  Saturation2/1 -> Sum7/1
  Saturation1/1 -> Rate Limiter/1
  RotSpeed/1 -> Sum2/2
  Sum8/1 -> Saturation1/1
  Gain5/1 -> Integrator1/1
  Integrator1/1 -> Sum8/2
  Sum2/1 -> Gain5/1, Gain6/1
  Compare To Constant1/1 -> Divide4/1
  Saturation/1 -> Sum2/1
  Rate Limiter/1 -> GenTorq/1
  2/1 -> Divide4/2, Compare To Constant1/1
  Divide4/1 -> Sum7/2, Scope2/1
  Sum7/1 -> Saturation/1
  WindSpeed/1 -> Optimall TSR / Radius/1
  Gain6/1 -> Sum8/1

== system LoFT_Example3/FOWT System/Subsystem1/FOWT10/Aerodynamics and Local Control Systems/Local Control Systems/Subsystem1 ==
  RotSpeed : Inport
  WindSpeed : Inport  Port=2
  3 : Inport  Port=3
  Nacelle Speed : Inport  Port=4
  1-D Lookup Table : Lookup_n-D  NumberOfTableDimensions=1  BreakpointsForDimension1=Controller.R.PS_WindSpeeds  Table=Controller.R.PS_BldPitchMin  InternalRulePriority=Speed  RndMeth=Simplest
  Compare To Constant : simulink/Logic and Bit Operations/Compare To Constant  relop=<=  const=0  OutDataTypeStr=boolean
  Constant : Constant  Value=7.55*pi/30
  Constant1 : Constant  Value=90*pi/180
  Delay : Delay  DelayLength=1  InitialCondition=0
  Divide3 : Product  Inputs=**
  Gain : Gain  Gain=Controller.KV *0.5
  Gain Scheduling : Subsystem
  Gain1 : Gain
  Rate Limiter : RateLimiter  RisingSlewLimit=2*pi/180  FallingSlewLimit=-2 * pi/180  SampleTimeMode=inherited
  Saturation : Saturate  UpperLimit=7.55*pi/30  LowerLimit=5*pi/30
  Saturation Dynamic : simulink/Discontinuities/Saturation Dynamic  OutMin=[]  OutMax=[]  OutDataTypeStr=Inherit: Same as second input  OutDataType=fixdt(1, 16)  OutScaling=2^-10  DoSatur=off
  Scope2 : Scope
  Sum1 : Sum  Inputs=|++
  Sum3 : Sum  Inputs=|+-
  Sum4 : Sum  Inputs=|+-
  BldPitch : Outport
  wires:
  Divide3/1 -> Sum4/2
  Sum3/1 -> Gain Scheduling/1(In1)
  Saturation Dynamic/1 -> Rate Limiter/1, Delay/1
  Compare To Constant/1 -> Divide3/1
  Constant/1 -> Sum4/1
  Constant1/1 -> Saturation Dynamic/1
  3/1 -> Compare To Constant/1, Divide3/2
  Delay/1 -> Gain Scheduling/3(In2)
  RotSpeed/1 -> Sum3/2
  Gain Scheduling/1(Out1) -> Sum1/1
  Sum1/1 -> Saturation Dynamic/2
  Gain/1 -> Sum1/2
  Nacelle Speed/1 -> Gain/1
  WindSpeed/1 -> 1-D Lookup Table/1  "Vhat"
  1-D Lookup Table/1 -> Gain1/1
  Gain1/1 -> Saturation Dynamic/3, Gain Scheduling/2(In3), Scope2/1
  Rate Limiter/1 -> BldPitch/1
  Sum4/1 -> Saturation/1
  Saturation/1 -> Sum3/1

== system LoFT_Example3/FOWT System/Subsystem1/FOWT10/Aerodynamics and Local Control Systems/Local Control Systems/Subsystem2 ==
  GenTorq : Inport
  BldPitch : Inport  Port=2
  Constant3 : Constant  Value=-Controller.torqueMax
  Gain 1 : Gain  Gain=Controller.SPS_kb/deg2rad(30)
  Gain 2 : Gain  Gain=Controller.omegaMax
  Gain 3 : Gain  Gain=-Controller.SPS_kt/Controller.torqueMax
  Sum5 : Sum  Inputs=|+-
  Sum6 : Sum  Inputs=|+-
  Delta_omega_g : Outport
  wires:
  Sum6/1 -> Gain 2/1
  Gain 1/1 -> Sum6/1
  Constant3/1 -> Sum5/2
  Gain 3/1 -> Sum6/2
  Sum5/1 -> Gain 3/1
  Gain 2/1 -> Delta_omega_g/1
  BldPitch/1 -> Gain 1/1
  GenTorq/1 -> Sum5/1

== system LoFT_Example3/FOWT System/Subsystem1/FOWT10/Aerodynamics and Local Control Systems/Local Control Systems/wind speed estimator ==
  In1 : Inport
  Discrete Filter : DiscreteFilter  Numerator=Controller.F.Wind.b  Denominator=Controller.F.Wind.a  InitialStates=2000
  Out1 : Outport
  wires:
  Discrete Filter/1 -> Out1/1
  In1/1 -> Discrete Filter/1

== system LoFT_Example3/FOWT System/Subsystem1/FOWT2/Aerodynamics and Local Control Systems/Local Control Systems/Subsystem ==
  WindSpeed : Inport
  2 : Inport  Port=2
  RotSpeed : Inport  Port=3
  Compare To Constant1 : simulink/Logic and Bit Operations/Compare To Constant  relop=>=  const=0  OutDataTypeStr=boolean
  Divide4 : Product  Inputs=**
  Gain5 : Gain  Gain=Controller.R.VS_KI
  Gain6 : Gain  Gain=Controller.R.VS_KP
  Integrator1 : Integrator  InitialCondition=Controller.torqueMax * 0.7  LimitOutput=on  UpperSaturationLimit=Controller.torqueMax
  Optimall TSR / Radius : Gain  Gain=Controller.R.VS_TSRopt/Controller.R.RotorRad
  Rate Limiter : RateLimiter  RisingSlewLimit=Controller.torqueMaxRate  FallingSlewLimit=-Controller.torqueMaxRate  SampleTimeMode=inherited
  Saturation : Saturate  UpperLimit=7.55*pi/30  LowerLimit=5*pi/30
  Saturation1 : Saturate  UpperLimit=Controller.torqueMax  LowerLimit=0
  Saturation2 : Saturate  UpperLimit=7.55*pi/30  LowerLimit=5*pi/30
  Scope2 : Scope
  Sum2 : Sum  Inputs=|+-
  Sum7 : Sum  Inputs=|+-
  Sum8 : Sum  Inputs=|++
  GenTorq : Outport
  wires:
  Optimall TSR / Radius/1 -> Saturation2/1
  Saturation2/1 -> Sum7/1
  Saturation1/1 -> Rate Limiter/1
  RotSpeed/1 -> Sum2/2
  Sum8/1 -> Saturation1/1
  Gain5/1 -> Integrator1/1
  Integrator1/1 -> Sum8/2
  Sum2/1 -> Gain5/1, Gain6/1
  Compare To Constant1/1 -> Divide4/1
  Saturation/1 -> Sum2/1
  Rate Limiter/1 -> GenTorq/1
  2/1 -> Divide4/2, Compare To Constant1/1
  Divide4/1 -> Sum7/2, Scope2/1
  Sum7/1 -> Saturation/1
  WindSpeed/1 -> Optimall TSR / Radius/1
  Gain6/1 -> Sum8/1

== system LoFT_Example3/FOWT System/Subsystem1/FOWT2/Aerodynamics and Local Control Systems/Local Control Systems/Subsystem1 ==
  RotSpeed : Inport
  WindSpeed : Inport  Port=2
  3 : Inport  Port=3
  Nacelle Speed : Inport  Port=4
  1-D Lookup Table : Lookup_n-D  NumberOfTableDimensions=1  BreakpointsForDimension1=Controller.R.PS_WindSpeeds  Table=Controller.R.PS_BldPitchMin  InternalRulePriority=Speed  RndMeth=Simplest
  Compare To Constant : simulink/Logic and Bit Operations/Compare To Constant  relop=<=  const=0  OutDataTypeStr=boolean
  Constant : Constant  Value=7.55*pi/30
  Constant1 : Constant  Value=90*pi/180
  Delay : Delay  DelayLength=1  InitialCondition=0
  Divide3 : Product  Inputs=**
  Gain : Gain  Gain=Controller.KV *0.5
  Gain Scheduling : Subsystem
  Gain1 : Gain
  Rate Limiter : RateLimiter  RisingSlewLimit=2*pi/180  FallingSlewLimit=-2 * pi/180  SampleTimeMode=inherited
  Saturation : Saturate  UpperLimit=7.55*pi/30  LowerLimit=5*pi/30
  Saturation Dynamic : simulink/Discontinuities/Saturation Dynamic  OutMin=[]  OutMax=[]  OutDataTypeStr=Inherit: Same as second input  OutDataType=fixdt(1, 16)  OutScaling=2^-10  DoSatur=off
  Scope2 : Scope
  Sum1 : Sum  Inputs=|++
  Sum3 : Sum  Inputs=|+-
  Sum4 : Sum  Inputs=|+-
  BldPitch : Outport
  wires:
  Divide3/1 -> Sum4/2
  Sum3/1 -> Gain Scheduling/1(In1)
  Saturation Dynamic/1 -> Rate Limiter/1, Delay/1
  Compare To Constant/1 -> Divide3/1
  Constant/1 -> Sum4/1
  Constant1/1 -> Saturation Dynamic/1
  3/1 -> Compare To Constant/1, Divide3/2
  Delay/1 -> Gain Scheduling/3(In2)
  RotSpeed/1 -> Sum3/2
  Gain Scheduling/1(Out1) -> Sum1/1
  Sum1/1 -> Saturation Dynamic/2
  Gain/1 -> Sum1/2
  Nacelle Speed/1 -> Gain/1
  WindSpeed/1 -> 1-D Lookup Table/1  "Vhat"
  1-D Lookup Table/1 -> Gain1/1
  Gain1/1 -> Saturation Dynamic/3, Gain Scheduling/2(In3), Scope2/1
  Rate Limiter/1 -> BldPitch/1
  Sum4/1 -> Saturation/1
  Saturation/1 -> Sum3/1

== system LoFT_Example3/FOWT System/Subsystem1/FOWT2/Aerodynamics and Local Control Systems/Local Control Systems/Subsystem2 ==
  GenTorq : Inport
  BldPitch : Inport  Port=2
  Constant3 : Constant  Value=-Controller.torqueMax
  Gain 1 : Gain  Gain=Controller.SPS_kb/deg2rad(30)
  Gain 2 : Gain  Gain=Controller.omegaMax
  Gain 3 : Gain  Gain=-Controller.SPS_kt/Controller.torqueMax
  Sum5 : Sum  Inputs=|+-
  Sum6 : Sum  Inputs=|+-
  Delta_omega_g : Outport
  wires:
  Sum6/1 -> Gain 2/1
  Gain 1/1 -> Sum6/1
  Constant3/1 -> Sum5/2
  Gain 3/1 -> Sum6/2
  Sum5/1 -> Gain 3/1
  Gain 2/1 -> Delta_omega_g/1
  BldPitch/1 -> Gain 1/1
  GenTorq/1 -> Sum5/1

== system LoFT_Example3/FOWT System/Subsystem1/FOWT2/Aerodynamics and Local Control Systems/Local Control Systems/wind speed estimator ==
  In1 : Inport
  Discrete Filter : DiscreteFilter  Numerator=Controller.F.Wind.b  Denominator=Controller.F.Wind.a  InitialStates=2000
  Out1 : Outport
  wires:
  Discrete Filter/1 -> Out1/1
  In1/1 -> Discrete Filter/1

== system LoFT_Example3/FOWT System/Subsystem1/FOWT3/Aerodynamics and Local Control Systems/Local Control Systems/Subsystem ==
  WindSpeed : Inport
  2 : Inport  Port=2
  RotSpeed : Inport  Port=3
  Compare To Constant1 : simulink/Logic and Bit Operations/Compare To Constant  relop=>=  const=0  OutDataTypeStr=boolean
  Divide4 : Product  Inputs=**
  Gain5 : Gain  Gain=Controller.R.VS_KI
  Gain6 : Gain  Gain=Controller.R.VS_KP
  Integrator1 : Integrator  InitialCondition=Controller.torqueMax * 0.7  LimitOutput=on  UpperSaturationLimit=Controller.torqueMax
  Optimall TSR / Radius : Gain  Gain=Controller.R.VS_TSRopt/Controller.R.RotorRad
  Rate Limiter : RateLimiter  RisingSlewLimit=Controller.torqueMaxRate  FallingSlewLimit=-Controller.torqueMaxRate  SampleTimeMode=inherited
  Saturation : Saturate  UpperLimit=7.55*pi/30  LowerLimit=5*pi/30
  Saturation1 : Saturate  UpperLimit=Controller.torqueMax  LowerLimit=0
  Saturation2 : Saturate  UpperLimit=7.55*pi/30  LowerLimit=5*pi/30
  Scope2 : Scope
  Sum2 : Sum  Inputs=|+-
  Sum7 : Sum  Inputs=|+-
  Sum8 : Sum  Inputs=|++
  GenTorq : Outport
  wires:
  Gain6/1 -> Sum8/1
  WindSpeed/1 -> Optimall TSR / Radius/1
  Sum7/1 -> Saturation/1
  Divide4/1 -> Scope2/1, Sum7/2
  2/1 -> Compare To Constant1/1, Divide4/2
  Rate Limiter/1 -> GenTorq/1
  Saturation/1 -> Sum2/1
  Compare To Constant1/1 -> Divide4/1
  Sum2/1 -> Gain6/1, Gain5/1
  Integrator1/1 -> Sum8/2
  Gain5/1 -> Integrator1/1
  Sum8/1 -> Saturation1/1
  RotSpeed/1 -> Sum2/2
  Saturation1/1 -> Rate Limiter/1
  Saturation2/1 -> Sum7/1
  Optimall TSR / Radius/1 -> Saturation2/1

== system LoFT_Example3/FOWT System/Subsystem1/FOWT3/Aerodynamics and Local Control Systems/Local Control Systems/Subsystem1 ==
  RotSpeed : Inport
  WindSpeed : Inport  Port=2
  3 : Inport  Port=3
  Nacelle Speed : Inport  Port=4
  1-D Lookup Table : Lookup_n-D  NumberOfTableDimensions=1  BreakpointsForDimension1=Controller.R.PS_WindSpeeds  Table=Controller.R.PS_BldPitchMin  InternalRulePriority=Speed  RndMeth=Simplest
  Compare To Constant : simulink/Logic and Bit Operations/Compare To Constant  relop=<=  const=0  OutDataTypeStr=boolean
  Constant : Constant  Value=7.55*pi/30
  Constant1 : Constant  Value=90*pi/180
  Delay : Delay  DelayLength=1  InitialCondition=0
  Divide3 : Product  Inputs=**
  Gain : Gain  Gain=Controller.KV *0.5
  Gain Scheduling : Subsystem
  Gain1 : Gain
  Rate Limiter : RateLimiter  RisingSlewLimit=2*pi/180  FallingSlewLimit=-2 * pi/180  SampleTimeMode=inherited
  Saturation : Saturate  UpperLimit=7.55*pi/30  LowerLimit=5*pi/30
  Saturation Dynamic : simulink/Discontinuities/Saturation Dynamic  OutMin=[]  OutMax=[]  OutDataTypeStr=Inherit: Same as second input  OutDataType=fixdt(1, 16)  OutScaling=2^-10  DoSatur=off
  Scope2 : Scope
  Sum1 : Sum  Inputs=|++
  Sum3 : Sum  Inputs=|+-
  Sum4 : Sum  Inputs=|+-
  BldPitch : Outport
  wires:
  Saturation/1 -> Sum3/1
  Sum4/1 -> Saturation/1
  Rate Limiter/1 -> BldPitch/1
  Gain1/1 -> Scope2/1, Gain Scheduling/2(In3), Saturation Dynamic/3
  1-D Lookup Table/1 -> Gain1/1
  WindSpeed/1 -> 1-D Lookup Table/1  "Vhat"
  Nacelle Speed/1 -> Gain/1
  Gain/1 -> Sum1/2
  Sum1/1 -> Saturation Dynamic/2
  Gain Scheduling/1(Out1) -> Sum1/1
  RotSpeed/1 -> Sum3/2
  Delay/1 -> Gain Scheduling/3(In2)
  3/1 -> Divide3/2, Compare To Constant/1
  Constant1/1 -> Saturation Dynamic/1
  Constant/1 -> Sum4/1
  Compare To Constant/1 -> Divide3/1
  Saturation Dynamic/1 -> Delay/1, Rate Limiter/1
  Sum3/1 -> Gain Scheduling/1(In1)
  Divide3/1 -> Sum4/2

== system LoFT_Example3/FOWT System/Subsystem1/FOWT3/Aerodynamics and Local Control Systems/Local Control Systems/Subsystem2 ==
  GenTorq : Inport
  BldPitch : Inport  Port=2
  Constant3 : Constant  Value=-Controller.torqueMax
  Gain 1 : Gain  Gain=Controller.SPS_kb/deg2rad(30)
  Gain 2 : Gain  Gain=Controller.omegaMax
  Gain 3 : Gain  Gain=-Controller.SPS_kt/Controller.torqueMax
  Sum5 : Sum  Inputs=|+-
  Sum6 : Sum  Inputs=|+-
  Delta_omega_g : Outport
  wires:
  GenTorq/1 -> Sum5/1
  BldPitch/1 -> Gain 1/1
  Gain 2/1 -> Delta_omega_g/1
  Sum5/1 -> Gain 3/1
  Gain 3/1 -> Sum6/2
  Constant3/1 -> Sum5/2
  Gain 1/1 -> Sum6/1
  Sum6/1 -> Gain 2/1

== system LoFT_Example3/FOWT System/Subsystem1/FOWT3/Aerodynamics and Local Control Systems/Local Control Systems/wind speed estimator ==
  In1 : Inport
  Discrete Filter : DiscreteFilter  Numerator=Controller.F.Wind.b  Denominator=Controller.F.Wind.a  InitialStates=2000
  Out1 : Outport
  wires:
  In1/1 -> Discrete Filter/1
  Discrete Filter/1 -> Out1/1

== system LoFT_Example3/FOWT System/Subsystem1/FOWT4/Aerodynamics and Local Control Systems/Local Control Systems/Subsystem ==
  WindSpeed : Inport
  2 : Inport  Port=2
  RotSpeed : Inport  Port=3
  Compare To Constant1 : simulink/Logic and Bit Operations/Compare To Constant  relop=>=  const=0  OutDataTypeStr=boolean
  Divide4 : Product  Inputs=**
  Gain5 : Gain  Gain=Controller.R.VS_KI
  Gain6 : Gain  Gain=Controller.R.VS_KP
  Integrator1 : Integrator  InitialCondition=Controller.torqueMax * 0.7  LimitOutput=on  UpperSaturationLimit=Controller.torqueMax
  Optimall TSR / Radius : Gain  Gain=Controller.R.VS_TSRopt/Controller.R.RotorRad
  Rate Limiter : RateLimiter  RisingSlewLimit=Controller.torqueMaxRate  FallingSlewLimit=-Controller.torqueMaxRate  SampleTimeMode=inherited
  Saturation : Saturate  UpperLimit=7.55*pi/30  LowerLimit=5*pi/30
  Saturation1 : Saturate  UpperLimit=Controller.torqueMax  LowerLimit=0
  Saturation2 : Saturate  UpperLimit=7.55*pi/30  LowerLimit=5*pi/30
  Scope2 : Scope
  Sum2 : Sum  Inputs=|+-
  Sum7 : Sum  Inputs=|+-
  Sum8 : Sum  Inputs=|++
  GenTorq : Outport
  wires:
  Optimall TSR / Radius/1 -> Saturation2/1
  Saturation2/1 -> Sum7/1
  Saturation1/1 -> Rate Limiter/1
  RotSpeed/1 -> Sum2/2
  Sum8/1 -> Saturation1/1
  Gain5/1 -> Integrator1/1
  Integrator1/1 -> Sum8/2
  Sum2/1 -> Gain5/1, Gain6/1
  Compare To Constant1/1 -> Divide4/1
  Saturation/1 -> Sum2/1
  Rate Limiter/1 -> GenTorq/1
  2/1 -> Divide4/2, Compare To Constant1/1
  Divide4/1 -> Sum7/2, Scope2/1
  Sum7/1 -> Saturation/1
  WindSpeed/1 -> Optimall TSR / Radius/1
  Gain6/1 -> Sum8/1

== system LoFT_Example3/FOWT System/Subsystem1/FOWT4/Aerodynamics and Local Control Systems/Local Control Systems/Subsystem1 ==
  RotSpeed : Inport
  WindSpeed : Inport  Port=2
  3 : Inport  Port=3
  Nacelle Speed : Inport  Port=4
  1-D Lookup Table : Lookup_n-D  NumberOfTableDimensions=1  BreakpointsForDimension1=Controller.R.PS_WindSpeeds  Table=Controller.R.PS_BldPitchMin  InternalRulePriority=Speed  RndMeth=Simplest
  Compare To Constant : simulink/Logic and Bit Operations/Compare To Constant  relop=<=  const=0  OutDataTypeStr=boolean
  Constant : Constant  Value=7.55*pi/30
  Constant1 : Constant  Value=90*pi/180
  Delay : Delay  DelayLength=1  InitialCondition=0
  Divide3 : Product  Inputs=**
  Gain : Gain  Gain=Controller.KV *0.5
  Gain Scheduling : Subsystem
  Gain1 : Gain
  Rate Limiter : RateLimiter  RisingSlewLimit=2*pi/180  FallingSlewLimit=-2 * pi/180  SampleTimeMode=inherited
  Saturation : Saturate  UpperLimit=7.55*pi/30  LowerLimit=5*pi/30
  Saturation Dynamic : simulink/Discontinuities/Saturation Dynamic  OutMin=[]  OutMax=[]  OutDataTypeStr=Inherit: Same as second input  OutDataType=fixdt(1, 16)  OutScaling=2^-10  DoSatur=off
  Scope2 : Scope
  Sum1 : Sum  Inputs=|++
  Sum3 : Sum  Inputs=|+-
  Sum4 : Sum  Inputs=|+-
  BldPitch : Outport
  wires:
  Divide3/1 -> Sum4/2
  Sum3/1 -> Gain Scheduling/1(In1)
  Saturation Dynamic/1 -> Rate Limiter/1, Delay/1
  Compare To Constant/1 -> Divide3/1
  Constant/1 -> Sum4/1
  Constant1/1 -> Saturation Dynamic/1
  3/1 -> Compare To Constant/1, Divide3/2
  Delay/1 -> Gain Scheduling/3(In2)
  RotSpeed/1 -> Sum3/2
  Gain Scheduling/1(Out1) -> Sum1/1
  Sum1/1 -> Saturation Dynamic/2
  Gain/1 -> Sum1/2
  Nacelle Speed/1 -> Gain/1
  WindSpeed/1 -> 1-D Lookup Table/1  "Vhat"
  1-D Lookup Table/1 -> Gain1/1
  Gain1/1 -> Saturation Dynamic/3, Gain Scheduling/2(In3), Scope2/1
  Rate Limiter/1 -> BldPitch/1
  Sum4/1 -> Saturation/1
  Saturation/1 -> Sum3/1

== system LoFT_Example3/FOWT System/Subsystem1/FOWT4/Aerodynamics and Local Control Systems/Local Control Systems/Subsystem2 ==
  GenTorq : Inport
  BldPitch : Inport  Port=2
  Constant3 : Constant  Value=-Controller.torqueMax
  Gain 1 : Gain  Gain=Controller.SPS_kb/deg2rad(30)
  Gain 2 : Gain  Gain=Controller.omegaMax
  Gain 3 : Gain  Gain=-Controller.SPS_kt/Controller.torqueMax
  Sum5 : Sum  Inputs=|+-
  Sum6 : Sum  Inputs=|+-
  Delta_omega_g : Outport
  wires:
  Sum6/1 -> Gain 2/1
  Gain 1/1 -> Sum6/1
  Constant3/1 -> Sum5/2
  Gain 3/1 -> Sum6/2
  Sum5/1 -> Gain 3/1
  Gain 2/1 -> Delta_omega_g/1
  BldPitch/1 -> Gain 1/1
  GenTorq/1 -> Sum5/1

== system LoFT_Example3/FOWT System/Subsystem1/FOWT4/Aerodynamics and Local Control Systems/Local Control Systems/wind speed estimator ==
  In1 : Inport
  Discrete Filter : DiscreteFilter  Numerator=Controller.F.Wind.b  Denominator=Controller.F.Wind.a  InitialStates=2000
  Out1 : Outport
  wires:
  Discrete Filter/1 -> Out1/1
  In1/1 -> Discrete Filter/1

== system LoFT_Example3/FOWT System/Subsystem1/FOWT5/Aerodynamics and Local Control Systems/Local Control Systems/Subsystem ==
  WindSpeed : Inport
  2 : Inport  Port=2
  RotSpeed : Inport  Port=3
  Compare To Constant1 : simulink/Logic and Bit Operations/Compare To Constant  relop=>=  const=0  OutDataTypeStr=boolean
  Divide4 : Product  Inputs=**
  Gain5 : Gain  Gain=Controller.R.VS_KI
  Gain6 : Gain  Gain=Controller.R.VS_KP
  Integrator1 : Integrator  InitialCondition=Controller.torqueMax * 0.7  LimitOutput=on  UpperSaturationLimit=Controller.torqueMax
  Optimall TSR / Radius : Gain  Gain=Controller.R.VS_TSRopt/Controller.R.RotorRad
  Rate Limiter : RateLimiter  RisingSlewLimit=Controller.torqueMaxRate  FallingSlewLimit=-Controller.torqueMaxRate  SampleTimeMode=inherited
  Saturation : Saturate  UpperLimit=7.55*pi/30  LowerLimit=5*pi/30
  Saturation1 : Saturate  UpperLimit=Controller.torqueMax  LowerLimit=0
  Saturation2 : Saturate  UpperLimit=7.55*pi/30  LowerLimit=5*pi/30
  Scope2 : Scope
  Sum2 : Sum  Inputs=|+-
  Sum7 : Sum  Inputs=|+-
  Sum8 : Sum  Inputs=|++
  GenTorq : Outport
  wires:
  Gain6/1 -> Sum8/1
  WindSpeed/1 -> Optimall TSR / Radius/1
  Sum7/1 -> Saturation/1
  Divide4/1 -> Scope2/1, Sum7/2
  2/1 -> Compare To Constant1/1, Divide4/2
  Rate Limiter/1 -> GenTorq/1
  Saturation/1 -> Sum2/1
  Compare To Constant1/1 -> Divide4/1
  Sum2/1 -> Gain6/1, Gain5/1
  Integrator1/1 -> Sum8/2
  Gain5/1 -> Integrator1/1
  Sum8/1 -> Saturation1/1
  RotSpeed/1 -> Sum2/2
  Saturation1/1 -> Rate Limiter/1
  Saturation2/1 -> Sum7/1
  Optimall TSR / Radius/1 -> Saturation2/1

== system LoFT_Example3/FOWT System/Subsystem1/FOWT5/Aerodynamics and Local Control Systems/Local Control Systems/Subsystem1 ==
  RotSpeed : Inport
  WindSpeed : Inport  Port=2
  3 : Inport  Port=3
  Nacelle Speed : Inport  Port=4
  1-D Lookup Table : Lookup_n-D  NumberOfTableDimensions=1  BreakpointsForDimension1=Controller.R.PS_WindSpeeds  Table=Controller.R.PS_BldPitchMin  InternalRulePriority=Speed  RndMeth=Simplest
  Compare To Constant : simulink/Logic and Bit Operations/Compare To Constant  relop=<=  const=0  OutDataTypeStr=boolean
  Constant : Constant  Value=7.55*pi/30
  Constant1 : Constant  Value=90*pi/180
  Delay : Delay  DelayLength=1  InitialCondition=0
  Divide3 : Product  Inputs=**
  Gain : Gain  Gain=Controller.KV *0.5
  Gain Scheduling : Subsystem
  Gain1 : Gain
  Rate Limiter : RateLimiter  RisingSlewLimit=2*pi/180  FallingSlewLimit=-2 * pi/180  SampleTimeMode=inherited
  Saturation : Saturate  UpperLimit=7.55*pi/30  LowerLimit=5*pi/30
  Saturation Dynamic : simulink/Discontinuities/Saturation Dynamic  OutMin=[]  OutMax=[]  OutDataTypeStr=Inherit: Same as second input  OutDataType=fixdt(1, 16)  OutScaling=2^-10  DoSatur=off
  Scope2 : Scope
  Sum1 : Sum  Inputs=|++
  Sum3 : Sum  Inputs=|+-
  Sum4 : Sum  Inputs=|+-
  BldPitch : Outport
  wires:
  Saturation/1 -> Sum3/1
  Sum4/1 -> Saturation/1
  Rate Limiter/1 -> BldPitch/1
  Gain1/1 -> Scope2/1, Gain Scheduling/2(In3), Saturation Dynamic/3
  1-D Lookup Table/1 -> Gain1/1
  WindSpeed/1 -> 1-D Lookup Table/1  "Vhat"
  Nacelle Speed/1 -> Gain/1
  Gain/1 -> Sum1/2
  Sum1/1 -> Saturation Dynamic/2
  Gain Scheduling/1(Out1) -> Sum1/1
  RotSpeed/1 -> Sum3/2
  Delay/1 -> Gain Scheduling/3(In2)
  3/1 -> Divide3/2, Compare To Constant/1
  Constant1/1 -> Saturation Dynamic/1
  Constant/1 -> Sum4/1
  Compare To Constant/1 -> Divide3/1
  Saturation Dynamic/1 -> Delay/1, Rate Limiter/1
  Sum3/1 -> Gain Scheduling/1(In1)
  Divide3/1 -> Sum4/2

== system LoFT_Example3/FOWT System/Subsystem1/FOWT5/Aerodynamics and Local Control Systems/Local Control Systems/Subsystem2 ==
  GenTorq : Inport
  BldPitch : Inport  Port=2
  Constant3 : Constant  Value=-Controller.torqueMax
  Gain 1 : Gain  Gain=Controller.SPS_kb/deg2rad(30)
  Gain 2 : Gain  Gain=Controller.omegaMax
  Gain 3 : Gain  Gain=-Controller.SPS_kt/Controller.torqueMax
  Sum5 : Sum  Inputs=|+-
  Sum6 : Sum  Inputs=|+-
  Delta_omega_g : Outport
  wires:
  GenTorq/1 -> Sum5/1
  BldPitch/1 -> Gain 1/1
  Gain 2/1 -> Delta_omega_g/1
  Sum5/1 -> Gain 3/1
  Gain 3/1 -> Sum6/2
  Constant3/1 -> Sum5/2
  Gain 1/1 -> Sum6/1
  Sum6/1 -> Gain 2/1
